simulink model "simulation_with_sensors_sim"  (R2023b)
settings: Solver=VariableStepAuto  StartTime=0.0  StopTime=1000  RelTol=1e-3
values from neighbouring files (symbols this model uses):
  a = R_E+500*1e3    (= 6871000)    [Sensors.m]    (also in sim_with_sensors.m = 6851.22197053; simulation_with_sensors.m = 26584)
  A_313 = ( R_om * R_i * R_OM )'    [simulation_with_sensors.m]
  e = 0    [Sensors.m]    (also in sim_with_sensors.m = 0.00183012221618; simulation_with_sensors.m = 0.00023103)
  H0 = sqrt(g01^2+g11^2+h11^2)*1e-9    [sim_with_sensors.m]    (also in simulation_with_sensors.m)
  I = diag([I1 I2 I3])*1e-9    [sim_with_sensors.m]    (also in simulation_with_sensors.m = diag([100.09 25.1 91.6]))
  i = 1.699980862034725    (= 1.69998086203)    [sim_with_sensors.m]    (also in simulation_with_sensors.m = 0.9601)
  I_inv = inv(I)    [simulation_with_sensors.m]
  incl = deg2rad(11.5)    [sim_with_sensors.m]    (also in simulation_with_sensors.m)
  n = n+1    (= 1)    [Sensors.m]    (also in sim_with_sensors.m = sqrt(mu/a^3); simulation_with_sensors.m = sqrt(astroConstants(13) / a^3))
  omegaE = deg2rad(15)/3600    [sim_with_sensors.m]    (also in simulation_with_sensors.m)
  P = zeros(lenn,lenm)    [Sensors.m]
  s0 = zeros(3,1)    [sim_with_sensors.m]    (also in simulation_with_sensors.m = [0; 0; 0])
  tol = 1e-2    (= 0.01)    [simulation_with_sensors.m]
  w0 = [0.2; 0; 0.2]    [simulation_with_sensors.m]
undefined symbols (not defined in the file or in its folder): A, c1, magnitude, N, n_sun, onesM, onesV, r_Fskew, rho_d, rho_s
libraries: matrix_library x11, vrlib x9, simulink x3, dspmathops x1
(part 2 of 2)

== system simulation_with_sensors_sim/Kinematics/Kinematics 313/s_313 - A/R3_1 ==
  x : Inport
  Constant : Constant  Value=[0; 0; 1]
  Constant1 : Constant  Value=0
  Cos : Trigonometry  Operator=cos
  Gain : Gain  Gain=-1
  Matrix Concatenate : Concatenate  NumInputs=3  Mode=Multidimensional array  ConcatenateDimension=2
  Sin : Trigonometry
  Vector Concatenate : Concatenate  NumInputs=3
  Vector Concatenate1 : Concatenate  NumInputs=3
  R3 : Outport
  wires:
  Matrix Concatenate/1 -> R3/1
  Constant1/1 -> Vector Concatenate1/3, Vector Concatenate/3
  x/1 -> Cos/1, Sin/1
  Vector Concatenate1/1 -> Matrix Concatenate/2
  Gain/1 -> Vector Concatenate/2
  Constant/1 -> Matrix Concatenate/3
  Cos/1 -> Vector Concatenate/1, Vector Concatenate1/2
  Sin/1 -> Gain/1, Vector Concatenate1/1
  Vector Concatenate/1 -> Matrix Concatenate/1

== system simulation_with_sensors_sim/Kinematics/Kinematics 313/s_313 - A/R3_2 ==
  x : Inport
  Constant : Constant  Value=[0; 0; 1]
  Constant1 : Constant  Value=0
  Cos : Trigonometry  Operator=cos
  Gain : Gain  Gain=-1
  Matrix Concatenate : Concatenate  NumInputs=3  Mode=Multidimensional array  ConcatenateDimension=2
  Sin : Trigonometry
  Vector Concatenate : Concatenate  NumInputs=3
  Vector Concatenate1 : Concatenate  NumInputs=3
  R3 : Outport
  wires:
  Vector Concatenate/1 -> Matrix Concatenate/1
  Sin/1 -> Vector Concatenate1/1, Gain/1
  Cos/1 -> Vector Concatenate1/2, Vector Concatenate/1
  Constant/1 -> Matrix Concatenate/3
  Gain/1 -> Vector Concatenate/2
  Vector Concatenate1/1 -> Matrix Concatenate/2
  x/1 -> Sin/1, Cos/1
  Constant1/1 -> Vector Concatenate/3, Vector Concatenate1/3
  Matrix Concatenate/1 -> R3/1
